simulink model "ex2"  (R2020a)
settings: Solver=VariableStepAuto  StartTime=0.0  StopTime=10.0  RelTol=1e-3
undefined symbols (not defined in the file or in its folder): den_Grz, num_Grz

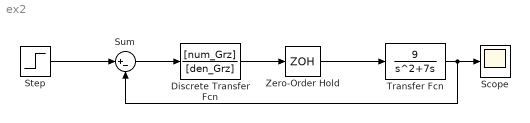
== system ex2 ==
  Discrete Transfer Fcn : DiscreteTransferFcn  Numerator=[num_Grz]  Denominator=[den_Grz]
  Scope : Scope
  Step : Step  SampleTime=0.1
  Sum : Sum  Inputs=|+-  SampleTime=0.1
  Transfer Fcn : TransferFcn  Numerator=[9]  Denominator=[1 7 0]
  Zero-Order Hold : ZeroOrderHold  SampleTime=-1
  wires:
  Step/1 -> Sum/1
  Sum/1 -> Discrete Transfer Fcn/1
  Discrete Transfer Fcn/1 -> Zero-Order Hold/1
  Zero-Order Hold/1 -> Transfer Fcn/1
  Transfer Fcn/1 -> Sum/2, Scope/1
